simulink model "filter2d1"  (Simulink 8.4)
settings: Solver=FixedStepDiscrete  SolverMode=SingleTasking  StartTime=0.0  StopTime=10.0  RelTol=1e-3
PreLoadFcn:
  | Param_filter
undefined symbols (not defined in the file or in its folder): Rec, SDTV
libraries: dspsigattribs x4, visionsinks x3, dspsigops x2, dspvision x1, visionfilter x1, visionconversions x1
settings Model: Creator=amatsumo  LastModifiedBy=kotsuka
settings DataIOCC: SaveOutput=off  SignalLogging=off  SaveTime=off
settings OptimizationCC: BlockReduction=off  ConditionallyExecuteInputs=off  InlineParams=on
settings DebuggingCC: AlgebraicLoopMsg=error  InheritedTsInSrcMsg=none  SingleTaskRateTransMsg=error
settings HardwareCC: ProdHWDeviceType=ASIC/FPGA->ASIC/FPGA  TargetLongLongMode=on  TargetIntDivRoundTo=Zero  TargetEndianess=LittleEndian  TargetHWDeviceType=MATLAB Host  ProdEqTarget=off

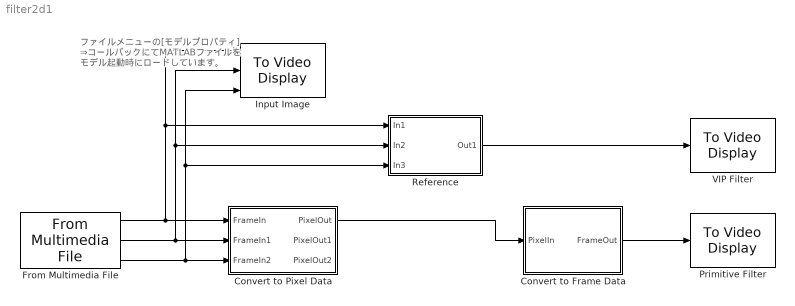
== system filter2d1 ==
  note: ファイルメニューの[モデルプロパティ]
      | ⇒コールバックにてMATLABファイルを
      | モデル起動時にロードしています。
  Convert to Frame Data : Subsystem
  Convert to Pixel Data : Subsystem
  From Multimedia File : dspvision/From Multimedia File  inputFilename=vipmen.avi  loop=on  numPlays=inf  outputStreams=Video only  videoDataType=uint8  audioDataType=int16  inheritSampleTime=off  userDefinedSampleTime=1/24  noAudioOutput=off  isIntensityVideo=off  fourcc=RGB  colorVideoFormat=Separate color signals  outputEOF=off  dataOrg=Column-major  audioFrameSize=1024  computeAudioFrameSize=off  outSamplingMode=Frame based
  Input Image : visionsinks/To Video Display  inputType=Obsolete  imagePorts=Separate color signals  OutputDevice=On-screen video monitor  fullScreen=off  videoWindowX=367  videoWindowY=50  saveWindowSize=off  videoWindowWidth=160  videoWindowHeight=120  dataOrg=Column-major  openAtMdlStart=on  isWindowOpen=on  inputColorFormat=RGB
  Primitive Filter : visionsinks/To Video Display  inputType=Obsolete  imagePorts=One multidimensional signal  OutputDevice=On-screen video monitor  fullScreen=off  videoWindowX=920  videoWindowY=48  saveWindowSize=off  videoWindowWidth=160  videoWindowHeight=120  dataOrg=Column-major  openAtMdlStart=on  isWindowOpen=on  inputColorFormat=RGB
  Reference : Subsystem
  VIP Filter : visionsinks/To Video Display  inputType=Obsolete  imagePorts=One multidimensional signal  OutputDevice=On-screen video monitor  fullScreen=off  videoWindowX=642  videoWindowY=48  saveWindowSize=off  videoWindowWidth=160  videoWindowHeight=120  dataOrg=Column-major  openAtMdlStart=on  isWindowOpen=on  inputColorFormat=RGB
  wires:
  From Multimedia File/1 -> Convert to Pixel Data/1(FrameIn), Input Image/1, Reference/1(In1)
  From Multimedia File/2 -> Convert to Pixel Data/2(FrameIn1), Input Image/2, Reference/2(In2)
  From Multimedia File/3 -> Convert to Pixel Data/3(FrameIn2), Input Image/3, Reference/3(In3)
  Reference/1(Out1) -> VIP Filter/1
  Convert to Frame Data/1(FrameOut) -> Primitive Filter/1
  Convert to Pixel Data/1(PixelOut) -> Convert to Frame Data/1(PixelIn)

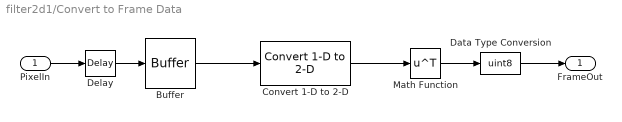
== system filter2d1/Convert to Frame Data ==
  PixelIn : Inport
  Buffer : Buffer  N=160*120
  Convert 1-D to 2-D : dspsigattribs/Convert 1-D to 2-D  M=160  N=120  frameBasedOut=off
  Data Type Conversion : DataTypeConversion  OutDataTypeStr=uint8  SaturateOnIntegerOverflow=on
  Delay : dspsigops/Delay  InputProcessing=Inherited (this choice will be removed - see release notes)  dly_unit=Samples  delay="0  %160-(2+1)"  ic_detail=off  dif_ic_for_ch=off  dif_ic_for_dly=off  ic=0  reset_popup=None
  Math Function : Math  Operator=transpose  SaturateOnIntegerOverflow=on
  FrameOut : Outport
  wires:
  Buffer/1 -> Convert 1-D to 2-D/1
  Convert 1-D to 2-D/1 -> Math Function/1
  PixelIn/1 -> Delay/1
  Math Function/1 -> Data Type Conversion/1
  Delay/1 -> Buffer/1
  Data Type Conversion/1 -> FrameOut/1

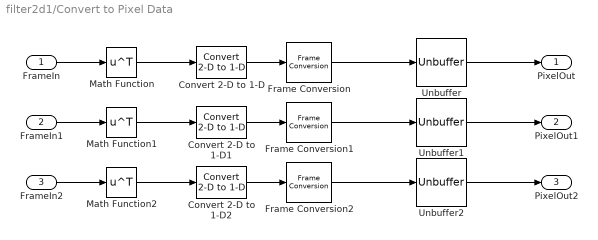
== system filter2d1/Convert to Pixel Data ==
  FrameIn : Inport
  FrameIn1 : Inport  Port=2
  FrameIn2 : Inport  Port=3
  Convert 2-D to 1-D : dspsigattribs/Convert 2-D to 1-D
  Convert 2-D to 1-D1 : dspsigattribs/Convert 2-D to 1-D
  Convert 2-D to 1-D2 : dspsigattribs/Convert 2-D to 1-D
  Frame Conversion : FrameConversion
  Frame Conversion1 : FrameConversion
  Frame Conversion2 : FrameConversion
  Math Function : Math  Operator=transpose  SaturateOnIntegerOverflow=on
  Math Function1 : Math  Operator=transpose  SaturateOnIntegerOverflow=on
  Math Function2 : Math  Operator=transpose  SaturateOnIntegerOverflow=on
  Unbuffer : Unbuffer
  Unbuffer1 : Unbuffer
  Unbuffer2 : Unbuffer
  PixelOut : Outport
  PixelOut1 : Outport  Port=2
  PixelOut2 : Outport  Port=3
  wires:
  Frame Conversion/1 -> Unbuffer/1
  Convert 2-D to 1-D/1 -> Frame Conversion/1
  FrameIn/1 -> Math Function/1
  Unbuffer/1 -> PixelOut/1
  Math Function/1 -> Convert 2-D to 1-D/1
  Frame Conversion1/1 -> Unbuffer1/1
  Convert 2-D to 1-D1/1 -> Frame Conversion1/1
  FrameIn1/1 -> Math Function1/1
  Unbuffer1/1 -> PixelOut1/1
  Math Function1/1 -> Convert 2-D to 1-D1/1
  Frame Conversion2/1 -> Unbuffer2/1
  Convert 2-D to 1-D2/1 -> Frame Conversion2/1
  FrameIn2/1 -> Math Function2/1
  Unbuffer2/1 -> PixelOut2/1
  Math Function2/1 -> Convert 2-D to 1-D2/1

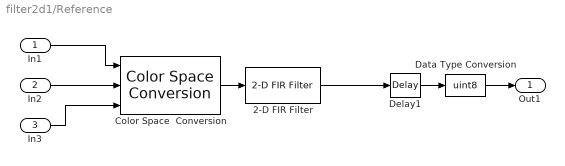
== system filter2d1/Reference ==
  In1 : Inport
  In2 : Inport  Port=2
  In3 : Inport  Port=3
  2-D FIR Filter : visionfilter/2-D FIR Filter  separable=off  filtSrc=Specify via dialog  filterMtrx=Hr  verticalFilter=[4 0]  horizontalFilter=[4 0]  outSize=Same as input port I  padType=Constant  padSrc=Specify via dialog  padVal=0  method=Convolution  firstCoeffMode=Binary point scaling  firstCoeffWordLength=7  firstCoeffFracLength=3  firstCoeffSignedness=Signed  firstCoeffDataTypeStr=fixdt(1,7,3)  firstCoeffLastDataTypeStr=fixdt(1,7,3)  firstCoeffMin=[]  firstCoeffMax=[]  outputMode=Binary point scaling  outputWordLength=19  outputFracLength=8  outputSignedness=Auto  outputDataTypeStr=fixdt([],19,8)  outputLastDataTypeStr=fixdt([],19,8)  outputMin=[]  outputMax=[]  accumDataTypeStr=Inherit: Same as product output  accumLastDataTypeStr=Inherit: Same as product output  prodOutputMode=Binary point scaling  prodOutputWordLength=15  prodOutputFracLength=3  prodOutputDataTypeStr=fixdt([],15,3)  prodOutputLastDataTypeStr=fixdt([],15,3)  roundingMode=Floor  overflowMode=on
  Color Space  Conversion : visionconversions/Color Space  Conversion  conversion=Obsolete  conversionActive=R'G'B' to intensity  wp_str=D65  rec=Rec. 601 (SDTV)  sys=1125/60/2:1  imagePorts=Separate color signals
  Data Type Conversion : DataTypeConversion  OutDataTypeStr=uint8  SaturateOnIntegerOverflow=on
  Delay1 : dspsigops/Delay  InputProcessing=Inherited (this choice will be removed - see release notes)  dly_unit=Samples  delay=1  ic_detail=off  dif_ic_for_ch=off  dif_ic_for_dly=off  ic=0  reset_popup=None
  Out1 : Outport
  wires:
  Data Type Conversion/1 -> Out1/1
  2-D FIR Filter/1 -> Delay1/1
  Delay1/1 -> Data Type Conversion/1
  In1/1 -> Color Space  Conversion/1
  In2/1 -> Color Space  Conversion/2
  In3/1 -> Color Space  Conversion/3
  Color Space  Conversion/1 -> 2-D FIR Filter/1
